simulink model "pro3simulink"  (R2014a)
settings: Solver=ode45  StartTime=0.0  StopTime=10.0  RelTol=1e-3
libraries: powerlib_meascontrol x1, simulink x1
settings Model: Creator=Fifi  LastModifiedBy=Fifi

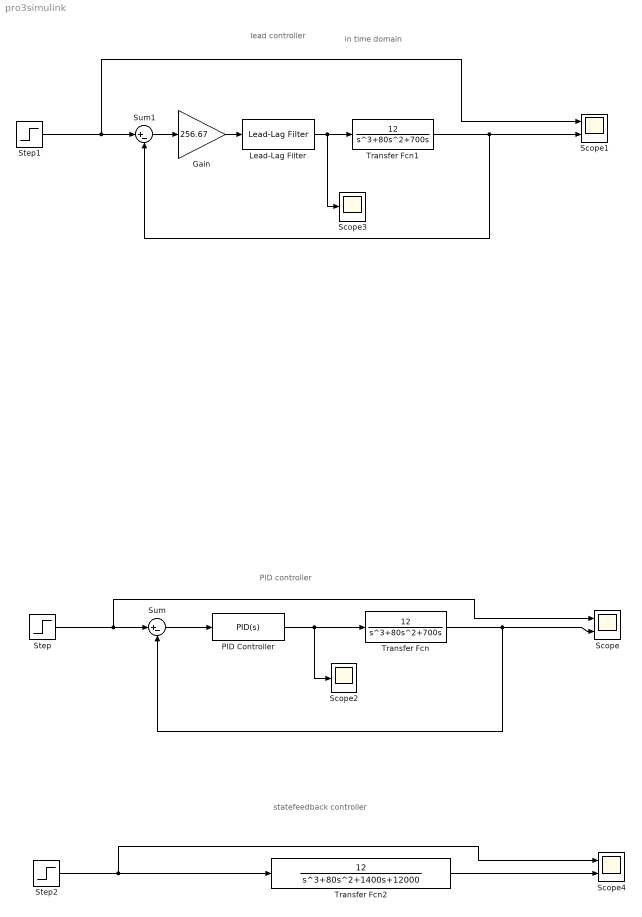
== system pro3simulink ==
  note: in time domain
  note: statefeedback controller
  note: PID controller
  note: lead controller
  Gain : Gain  Gain=256.67
  Lead-Lag Filter : powerlib_meascontrol/Filters/Lead-Lag Filter  T1=0.1  T2=0.067  Vdc_Init=0  Ts=0
  PID Controller : simulink/Continuous/PID Controller  Controller=PID  TimeDomain=Continuous-time  SampleTime=1  IntegratorMethod=Forward Euler  FilterMethod=Forward Euler  Form=Parallel  P=1424  I=503  D=124  N=200  InitialConditionSource=internal  InitialConditionForIntegrator=0  InitialConditionForFilter=0  ExternalReset=none  LimitOutput=off  UpperSaturationLimit=inf  LowerSaturationLimit=-inf  LinearizeAsGain=on  AntiWindupMode=none  Kb=1  TrackingMode=off  Kt=1  PParamMin=[]  PParamMax=[]  IParamMin=[]  IParamMax=[]  DParamMin=[]  DParamMax=[]  NParamMin=[]  NParamMax=[]  KbParamMin=[]  KbParamMax=[]  KtParamMin=[]  KtParamMax=[]  POutMin=[]  POutMax=[]  IOutMin=[]  IOutMax=[]  DOutMin=[]  DOutMax=[]  NOutMin=[]  NOutMax=[]  KbOutMin=[]  KbOutMax=[]  KtOutMin=[]  KtOutMax=[]  IntegratorOutMin=[]  IntegratorOutMax=[]  FilterOutMin=[]  FilterOutMax=[]  SumOutMin=[]  SumOutMax=[]  SumI1OutMin=[]  SumI1OutMax=[]  SumI2OutMin=[]  SumI2OutMax=[]  SumI3OutMin=[]  SumI3OutMax=[]  SumDOutMin=[]  SumDOutMax=[]  SaturationOutMin=[]  SaturationOutMax=[]  IntegratorContinuousStateAttributes=''  IntegratorStateMustResolveToSignalObject=off  IntegratorRTWStateStorageClass=Auto  FilterContinuousStateAttributes=''  FilterStateMustResolveToSignalObject=off  FilterRTWStateStorageClass=Auto
  Scope : Scope  NumInputPorts=2
      settings: TimeRange=10  YMin=0~-5  YMax=1.5~5
  Scope1 : Scope  NumInputPorts=2
      settings: TimeRange=10  YMin=0~-5  YMax=1.5~5
  Scope2 : Scope
      settings: TimeRange=10  YMin=0  YMax=1.5  SaveName=ScopeData2
  Scope3 : Scope
      settings: TimeRange=10  YMin=0  YMax=1.5  SaveName=ScopeData3
  Scope4 : Scope  NumInputPorts=2
      settings: TimeRange=10  YMin=0~-5  YMax=1.5~5  SaveName=ScopeData4
  Step : Step  SampleTime=0
  Step1 : Step  SampleTime=0
  Step2 : Step  SampleTime=0
  Sum : Sum  Inputs=|+-
  Sum1 : Sum  Inputs=|+-
  Transfer Fcn : TransferFcn  Numerator=[12]  Denominator=[1 80 700 0]
  Transfer Fcn1 : TransferFcn  Numerator=[12]  Denominator=[1 80 700 0]
  Transfer Fcn2 : TransferFcn  Numerator=[12]  Denominator=[1 80 1400 12000]
  wires:
  Step/1 -> Scope/1, Sum/1
  Sum/1 -> PID Controller/1
  Transfer Fcn/1 -> Scope/2, Sum/2
  PID Controller/1 -> Scope2/1, Transfer Fcn/1
  Step1/1 -> Scope1/1, Sum1/1
  Transfer Fcn1/1 -> Scope1/2, Sum1/2
  Lead-Lag Filter/1 -> Scope3/1, Transfer Fcn1/1
  Gain/1 -> Lead-Lag Filter/1
  Sum1/1 -> Gain/1
  Transfer Fcn2/1 -> Scope4/2
  Step2/1 -> Transfer Fcn2/1, Scope4/1
